simulink model "model_for_validation_bottom_section"  (R2022b)
settings: Solver=FixedStepAuto  StartTime=0.0  StopTime=5400  FixedStep=0.01  RelTol=1e-3
values from neighbouring files (symbols this model uses):
  A_bhp = area_cilinder    (= 0.006647610055)    [model_for_validation_bottom_section_script.m]
  A_bhp_air = A_thp_air    (= 0.0028902652413)    [model_for_validation_bottom_section_script.m]
  A_bi = area_cilinder    (= 0.006647610055)    [model_for_validation_bottom_section_script.m]
  A_bi_air = A_ti_air    (= 0.00578053048261)    [model_for_validation_bottom_section_script.m]
  A_bm = area_cilinder    (= 0.006647610055)    [model_for_validation_bottom_section_script.m]
  A_bm_air = A_tm_air    (= 0.0101159283446)    [model_for_validation_bottom_section_script.m]
  c_bc = c_tc    (= 460)    [model_for_validation_bottom_section_script.m]
  c_bhp = c_tm    (= 460)    [model_for_validation_bottom_section_script.m]
  c_bi = c_ti    (= 880)    [model_for_validation_bottom_section_script.m]
  c_bm = c_tm    (= 460)    [model_for_validation_bottom_section_script.m]
  D = 0    [model_for_validation_bottom_section_script.m]
  d_bhp = d_thp    (= 0.01)    [model_for_validation_bottom_section_script.m]
  d_bi = d_ti    (= 0.02)    [model_for_validation_bottom_section_script.m]
  d_bm = d_tm    (= 0.035)    [model_for_validation_bottom_section_script.m]
  h_c = 26.5    [model_for_validation_bottom_section_script.m]
  I = 0    [model_for_validation_bottom_section_script.m]
  k_bhp = k_tm    (= 22)    [model_for_validation_bottom_section_script.m]
  k_bi = k_ti    (= 0.3)    [model_for_validation_bottom_section_script.m]
  k_bm = k_tm    (= 22)    [model_for_validation_bottom_section_script.m]
  m_bc = m_tc    (= 0.0640332)    [model_for_validation_bottom_section_script.m]
  m_bhp = m_thp    (= 0.511865974235)    [model_for_validation_bottom_section_script.m]
  m_bi = m_ti    (= 0.29249484242)    [model_for_validation_bottom_section_script.m]
  m_bm = m_tm    (= 1.79153090982)    [model_for_validation_bottom_section_script.m]
  P = 100    [model_for_validation_bottom_section_script.m]
  P_rice = 1400    [model_for_validation_bottom_section_script.m]
  T_a = 18    [model_for_validation_bottom_section_script.m]
  T_init = T_a    (= 18)    [model_for_validation_bottom_section_script.m]
  T_setpoint = 285    [model_for_validation_bottom_section_script.m]
libraries: slpidlib x2, simulink x1
settings Model: PauseTimes=23  Creator=DLubbers  LastModifiedBy=DLubbers

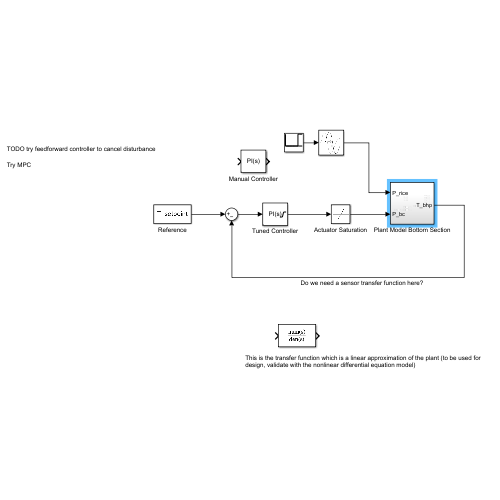
[thumbnail: Simulink's stored preview of the top-level diagram]
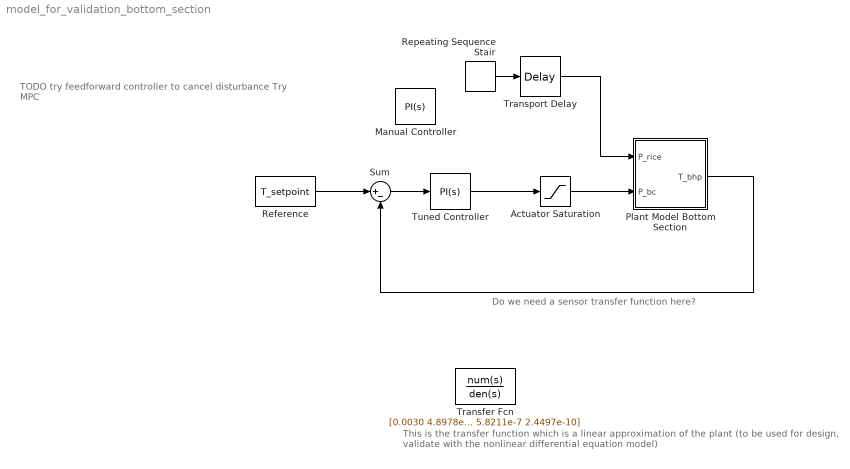
== system model_for_validation_bottom_section ==
  note: TODO try feedforward controller to cancel disturbance
      |
      | Try MPC
  note: This is the transfer function which is a linear approximation of the plant (to be used for design, validate with the nonlinear differential equation model)
  note: Do we need a sensor transfer function here?
  Actuator Saturation : Saturate  UpperLimit=690  LowerLimit=0
  Manual Controller : slpidlib/PID Controller  Controller=PI  Form=Parallel  TimeDomain=Continuous-time  UseExternalTs=off  SampleTime=-1  IntegratorMethod=Forward Euler  FilterMethod=Forward Euler  ControllerParametersSource=internal  P=P  I=I  UseKiTs=off  D=D  N=100  UseFilter=on  TunerSelectOption=Transfer Function Based (PID Tuner App)  InitialConditionSource=internal  InitialConditionForIntegrator=0  InitialConditionForFilter=0  DifferentiatorICPrevScaledInput=0  ExternalReset=none  TrackingMode=off  Kt=1  LimitOutput=off  SatLimitsSource=internal  UpperSaturationLimit=inf  LowerSaturationLimit=-inf  LinearizeAsGain=on  AntiWindupMode=none  Kb=1  LimitIntegrator=off  UpperIntegratorSaturationLimit=inf  LowerIntegratorSaturationLimit=-inf  POutMin=[]  POutMax=[]  IOutMin=[]  IOutMax=[]  DOutMin=[]  DOutMax=[]  NOutMin=[]  NOutMax=[]  SumOutMin=[]  SumOutMax=[]  SaturationOutMin=[]  SaturationOutMax=[]  PParamMin=[]  PParamMax=[]  IParamMin=[]  IParamMax=[]  DParamMin=[]  DParamMax=[]  NParamMin=[]  NParamMax=[]  KbParamMin=[]  KbParamMax=[]  KtParamMin=[]  KtParamMax=[]  KbOutMin=[]  KbOutMax=[]  KtOutMin=[]  KtOutMax=[]  IntegratorOutMin=[]  IntegratorOutMax=[]  FilterOutMin=[]  FilterOutMax=[]  SumI1OutMin=[]  SumI1OutMax=[]  SumI2OutMin=[]  SumI2OutMax=[]  SumI3OutMin=[]  SumI3OutMax=[]  SumI4OutMin=[]  SumI4OutMax=[]  SumDOutMin=[]  SumDOutMax=[]  DifferentiatorOutMin=[]  DifferentiatorOutMax=[]  FilterDiffOutCoefMin=[]  FilterDiffOutCoefMax=[]  ReciprocalOutMin=[]  ReciprocalOutMax=[]  SumDenOutMin=[]  SumDenOutMax=[]  SumNumOutMin=[]  SumNumOutMax=[]  DivideOutMin=[]  DivideOutMax=[]  UdiffTsProdOutMin=[]  UdiffTsProdOutMax=[]  NTsProdOutMin=[]  NTsProdOutMax=[]  UintegralTsProdOutMin=[]  UintegralTsProdOutMax=[]  UngainTsProdOutMin=[]  UngainTsProdOutMax=[]  ClampingZeroOutDataTypeStr=Inherit: Inherit via back propagation  ClampingZeroOutMin=[]  ClampingZeroOutMax=[]  FilterDenConstantOutDataTypeStr=Inherit: Inherit via back propagation  FilterDenConstantOutMin=[]  FilterDenConstantOutMax=[]  PCopyOutDataTypeStr=Inherit: Inherit via back propagation  PCopyOutMin=[]  PCopyOutMax=[]  NCopyOutDataTypeStr=Inherit: Inherit via back propagation  NCopyOutMin=[]  NCopyOutMax=[]  IntegratorContinuousStateAttributes=''  IntegratorStateMustResolveToSignalObject=off  IntegratorRTWStateStorageClass=Auto  FilterContinuousStateAttributes=''  FilterStateMustResolveToSignalObject=off  FilterRTWStateStorageClass=Auto  ParallelPVariant=InternalParameters  IdealPVariant=Disabled  IVariant=InternalParameters  DVariant=Disabled  IntegratorVariant=Continuous  SatVariant=Disabled  AWVariant=Passthrough  PCopyVariant=Disabled  TRVariant=Disabled  FdbkBlocksVariant=Forward  IdealPFdbkVariant=Disabled  SatFdbkVariant=Disabled  DerivativeFilterVariant=Disabled  NVariant=Disabled  NCopyVariant=Disabled_SignalSpec  FilterICVariant=Disabled  IntegratorICVariant=InternalICs  ExternalResetVariant=Disabled  TRSumVariant=Passthrough  SumFdbkVariant=Disabled  SumVariant=Sum_PI  TsampFilterVariant=InternalTs  TsampNgainVariant=Passthrough  TsampIntegralVariant=Passthrough  ExternalSaturationOutDataTypeStr=Inherit: Same as second input
  Plant Model Bottom Section : Subsystem
  Reference : Constant  Value=T_setpoint
  Repeating Sequence Stair : simulink/Sources/Repeating Sequence Stair  OutValues=[0 0 0 0 0 0 0 0 0 P_rice P_rice P_rice].'  tsamp=1  OutMin=[]  OutMax=[]  OutDataTypeStr=double  OutputDataTypeScalingMode=double  OutDataType=fixdt(0,8)  ConRadixGroup=Best Precision: Vector-wise  OutScaling=2^-12
  Sum : Sum  Inputs=|+-
  Transfer Fcn : TransferFcn  Numerator=[0.0030 4.8978e-5 2.5849e-7 4.3592e-10]  Denominator=[1 0.0288 2.3163e-4 5.8211e-7 2.4497e-10]
  Transport Delay : TransportDelay  DelayTime=3600
  Tuned Controller : slpidlib/PID Controller  Controller=PI  Form=Parallel  TimeDomain=Continuous-time  UseExternalTs=off  SampleTime=-1  IntegratorMethod=Forward Euler  FilterMethod=Forward Euler  ControllerParametersSource=internal  P=5.14299711444075  I=0.0389996474927596  UseKiTs=off  D=D  N=100  UseFilter=on  TunerSelectOption=Transfer Function Based (PID Tuner App)  InitialConditionSource=internal  InitialConditionForIntegrator=0  InitialConditionForFilter=0  DifferentiatorICPrevScaledInput=0  ExternalReset=none  TrackingMode=off  Kt=1  LimitOutput=on  SatLimitsSource=internal  UpperSaturationLimit=690  LowerSaturationLimit=0  LinearizeAsGain=on  AntiWindupMode=clamping  Kb=1  LimitIntegrator=off  UpperIntegratorSaturationLimit=inf  LowerIntegratorSaturationLimit=-inf  POutMin=[]  POutMax=[]  IOutMin=[]  IOutMax=[]  DOutMin=[]  DOutMax=[]  NOutMin=[]  NOutMax=[]  SumOutMin=[]  SumOutMax=[]  SaturationOutMin=[]  SaturationOutMax=[]  PParamMin=[]  PParamMax=[]  IParamMin=[]  IParamMax=[]  DParamMin=[]  DParamMax=[]  NParamMin=[]  NParamMax=[]  KbParamMin=[]  KbParamMax=[]  KtParamMin=[]  KtParamMax=[]  KbOutMin=[]  KbOutMax=[]  KtOutMin=[]  KtOutMax=[]  IntegratorOutMin=[]  IntegratorOutMax=[]  FilterOutMin=[]  FilterOutMax=[]  SumI1OutMin=[]  SumI1OutMax=[]  SumI2OutMin=[]  SumI2OutMax=[]  SumI3OutMin=[]  SumI3OutMax=[]  SumI4OutMin=[]  SumI4OutMax=[]  SumDOutMin=[]  SumDOutMax=[]  DifferentiatorOutMin=[]  DifferentiatorOutMax=[]  FilterDiffOutCoefMin=[]  FilterDiffOutCoefMax=[]  ReciprocalOutMin=[]  ReciprocalOutMax=[]  SumDenOutMin=[]  SumDenOutMax=[]  SumNumOutMin=[]  SumNumOutMax=[]  DivideOutMin=[]  DivideOutMax=[]  UdiffTsProdOutMin=[]  UdiffTsProdOutMax=[]  NTsProdOutMin=[]  NTsProdOutMax=[]  UintegralTsProdOutMin=[]  UintegralTsProdOutMax=[]  UngainTsProdOutMin=[]  UngainTsProdOutMax=[]  ClampingZeroOutDataTypeStr=Inherit: Inherit via back propagation  ClampingZeroOutMin=[]  ClampingZeroOutMax=[]  FilterDenConstantOutDataTypeStr=Inherit: Inherit via back propagation  FilterDenConstantOutMin=[]  FilterDenConstantOutMax=[]  PCopyOutDataTypeStr=Inherit: Inherit via back propagation  PCopyOutMin=[]  PCopyOutMax=[]  NCopyOutDataTypeStr=Inherit: Inherit via back propagation  NCopyOutMin=[]  NCopyOutMax=[]  IntegratorContinuousStateAttributes=''  IntegratorStateMustResolveToSignalObject=off  IntegratorRTWStateStorageClass=Auto  FilterContinuousStateAttributes=''  FilterStateMustResolveToSignalObject=off  FilterRTWStateStorageClass=Auto  ParallelPVariant=InternalParameters  IdealPVariant=Disabled  IVariant=InternalParameters  DVariant=Disabled  IntegratorVariant=Continuous  SatVariant=Enabled  AWVariant=ContClampingParallel  PCopyVariant=Disabled  TRVariant=Disabled  FdbkBlocksVariant=Forward  IdealPFdbkVariant=Disabled  SatFdbkVariant=Disabled  DerivativeFilterVariant=Disabled  NVariant=Disabled  NCopyVariant=Disabled_SignalSpec  FilterICVariant=Disabled  IntegratorICVariant=InternalICs  ExternalResetVariant=Disabled  TRSumVariant=Passthrough  SumFdbkVariant=Disabled  SumVariant=Sum_PI  TsampFilterVariant=InternalTs  TsampNgainVariant=Passthrough  TsampIntegralVariant=Passthrough  ExternalSaturationOutDataTypeStr=Inherit: Same as second input
  wires:
  Transport Delay/1 -> Plant Model Bottom Section/1(P_rice)
  Tuned Controller/1 -> Actuator Saturation/1
  Plant Model Bottom Section/1(T_bhp) -> Sum/2
  Sum/1 -> Tuned Controller/1
  Reference/1 -> Sum/1
  Actuator Saturation/1 -> Plant Model Bottom Section/2(P_bc)
  Repeating Sequence Stair/1 -> Transport Delay/1

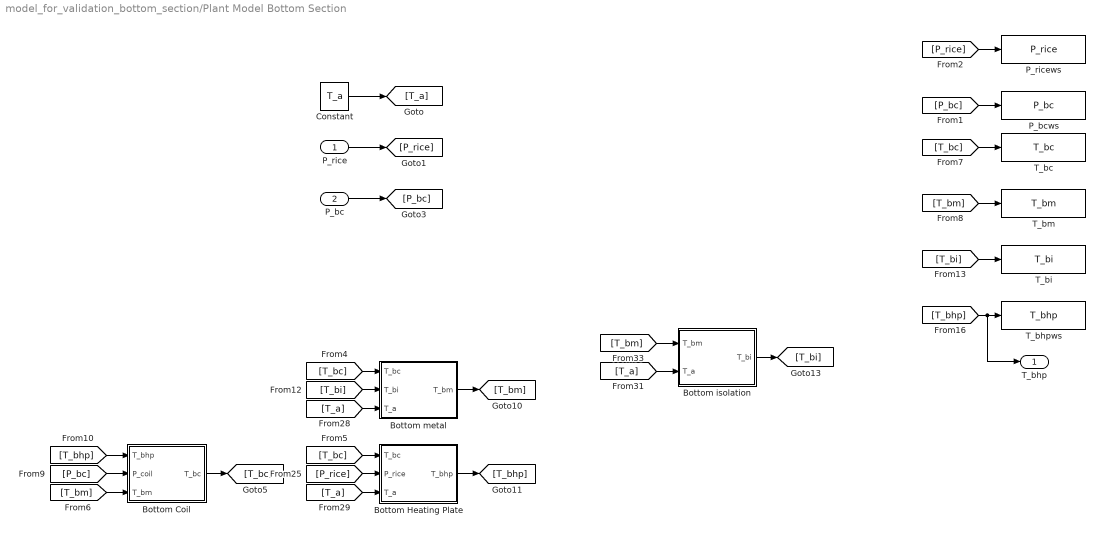
== system model_for_validation_bottom_section/Plant Model Bottom Section ==
  P_rice : Inport
  P_bc : Inport  Port=2
  Bottom Coil : Subsystem
  Bottom Heating Plate : Subsystem
  Bottom isolation : Subsystem
  Bottom metal : Subsystem
  Constant : Constant  Value=T_a
  P_bcws : ToWorkspace  VariableName=P_bc  SaveFormat=Timeseries  SampleTime=-1
  P_ricews : ToWorkspace  VariableName=P_rice  SaveFormat=Timeseries  SampleTime=-1
  T_bc : ToWorkspace  VariableName=T_bc  SaveFormat=Timeseries  SampleTime=-1
  T_bhpws : ToWorkspace  VariableName=T_bhp  SaveFormat=Timeseries  SampleTime=-1
  T_bi : ToWorkspace  VariableName=T_bi  SaveFormat=Timeseries  SampleTime=-1
  T_bm : ToWorkspace  VariableName=T_bm  SaveFormat=Timeseries  SampleTime=-1
  T_bhp : Outport
  wires:
  Constant/1 -> [T_a]
  [T_bhp] -> T_bhp/1, T_bhpws/1
  Bottom metal/1(T_bm) -> [T_bm]
  Bottom Coil/1(T_bc) -> [T_bc]
  [T_bc] -> Bottom metal/1(T_bc)
  [T_bi] -> T_bi/1
  [T_bm] -> Bottom isolation/1(T_bm)
  [T_a] -> Bottom Heating Plate/3(T_a)
  [T_a] -> Bottom metal/3(T_a)
  [T_bi] -> Bottom metal/2(T_bi)
  Bottom Heating Plate/1(T_bhp) -> [T_bhp]
  [T_bc] -> T_bc/1
  [T_a] -> Bottom isolation/2(T_a)
  [T_bhp] -> Bottom Coil/1(T_bhp)
  [T_bc] -> Bottom Heating Plate/1(T_bc)
  Bottom isolation/1(T_bi) -> [T_bi]
  [P_bc] -> Bottom Coil/2(P_coil)
  [P_rice] -> Bottom Heating Plate/2(P_rice)
  [T_bm] -> Bottom Coil/3(T_bm)
  [T_bm] -> T_bm/1
  P_bc/1 -> [P_bc]
  P_rice/1 -> [P_rice]
  [P_rice] -> P_ricews/1
  [P_bc] -> P_bcws/1

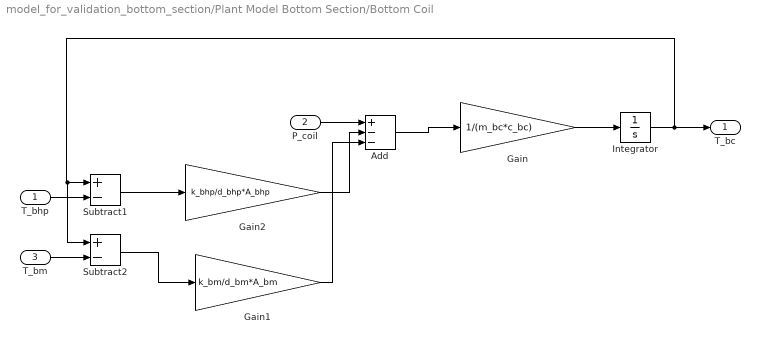
== system model_for_validation_bottom_section/Plant Model Bottom Section/Bottom Coil ==
  T_bhp : Inport
  P_coil : Inport  Port=2
  T_bm : Inport  Port=3
  Add : Sum  Inputs=+--
  Gain : Gain  Gain=1/(m_bc*c_bc)
  Gain1 : Gain  Gain=k_bm/d_bm*A_bm
  Gain2 : Gain  Gain=k_bhp/d_bhp*A_bhp
  Integrator : Integrator  InitialCondition=T_init
  Subtract1 : Sum  Inputs=+-
  Subtract2 : Sum  Inputs=+-
  T_bc : Outport
  wires:
  Gain/1 -> Integrator/1
  Add/1 -> Gain/1
  Subtract1/1 -> Gain2/1
  Gain2/1 -> Add/2
  T_bhp/1 -> Subtract1/2
  Integrator/1 -> T_bc/1, Subtract2/1, Subtract1/1
  P_coil/1 -> Add/1
  T_bm/1 -> Subtract2/2
  Subtract2/1 -> Gain1/1
  Gain1/1 -> Add/3

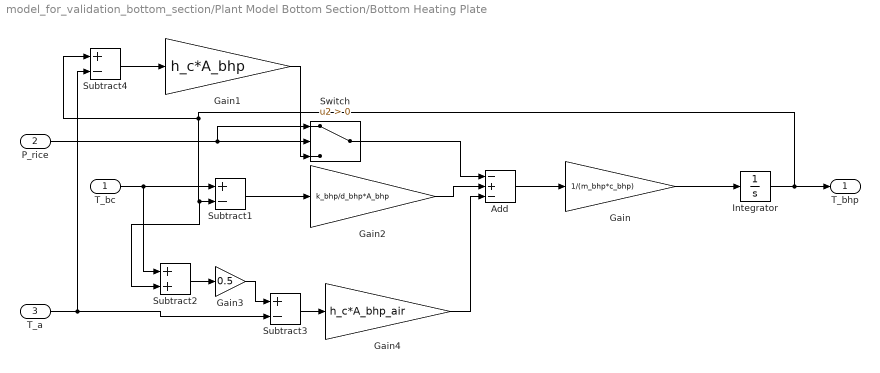
== system model_for_validation_bottom_section/Plant Model Bottom Section/Bottom Heating Plate ==
  T_bc : Inport
  P_rice : Inport  Port=2
  T_a : Inport  Port=3
  Add : Sum  Inputs=-+-
  Gain : Gain  Gain=1/(m_bhp*c_bhp)
  Gain1 : Gain  Gain=h_c*A_bhp
  Gain2 : Gain  Gain=k_bhp/d_bhp*A_bhp
  Gain3 : Gain  Gain=0.5
  Gain4 : Gain  Gain=h_c*A_bhp_air
  Integrator : Integrator  InitialCondition=T_init
  Subtract1 : Sum  Inputs=+-
  Subtract2 : Sum
  Subtract3 : Sum  Inputs=+-
  Subtract4 : Sum  Inputs=+-
  Switch : Switch  Criteria=u2 > Threshold  SaturateOnIntegerOverflow=off  InputSameDT=off
  T_bhp : Outport
  wires:
  P_rice/1 -> Switch/1, Switch/2
  Gain/1 -> Integrator/1
  Integrator/1 -> T_bhp/1, Subtract4/1, Subtract2/2, Subtract1/2
  Add/1 -> Gain/1
  Subtract1/1 -> Gain2/1
  T_bc/1 -> Subtract2/1, Subtract1/1
  Subtract3/1 -> Gain4/1
  T_a/1 -> Subtract4/2, Subtract3/2
  Subtract2/1 -> Gain3/1
  Gain3/1 -> Subtract3/1
  Gain2/1 -> Add/2
  Gain4/1 -> Add/3
  Switch/1 -> Add/1
  Gain1/1 -> Switch/3
  Subtract4/1 -> Gain1/1

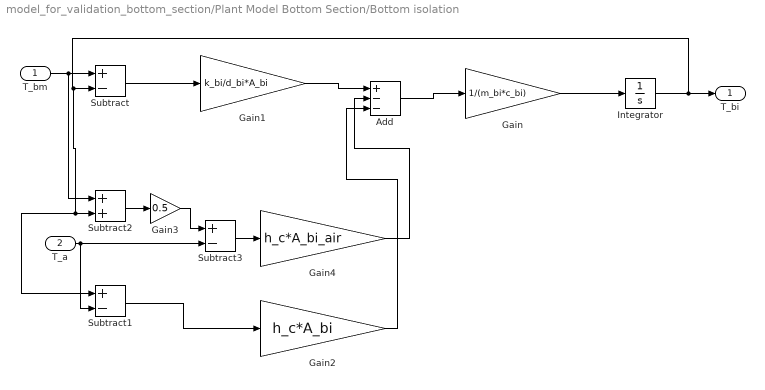
== system model_for_validation_bottom_section/Plant Model Bottom Section/Bottom isolation ==
  T_bm : Inport
  T_a : Inport  Port=2
  Add : Sum  Inputs=+--
  Gain : Gain  Gain=1/(m_bi*c_bi)
  Gain1 : Gain  Gain=k_bi/d_bi*A_bi
  Gain2 : Gain  Gain=h_c*A_bi
  Gain3 : Gain  Gain=0.5
  Gain4 : Gain  Gain=h_c*A_bi_air
  Integrator : Integrator  InitialCondition=T_init
  Subtract : Sum  Inputs=+-
  Subtract1 : Sum  Inputs=+-
  Subtract2 : Sum
  Subtract3 : Sum  Inputs=+-
  T_bi : Outport
  wires:
  Subtract/1 -> Gain1/1
  Gain/1 -> Integrator/1
  Add/1 -> Gain/1
  Integrator/1 -> Subtract2/2, Subtract1/1, Subtract/2, T_bi/1
  T_bm/1 -> Subtract2/1, Subtract/1
  Gain1/1 -> Add/1
  Subtract2/1 -> Gain3/1
  Gain3/1 -> Subtract3/1
  T_a/1 -> Subtract1/2, Subtract3/2
  Subtract3/1 -> Gain4/1
  Gain4/1 -> Add/2
  Gain2/1 -> Add/3
  Subtract1/1 -> Gain2/1

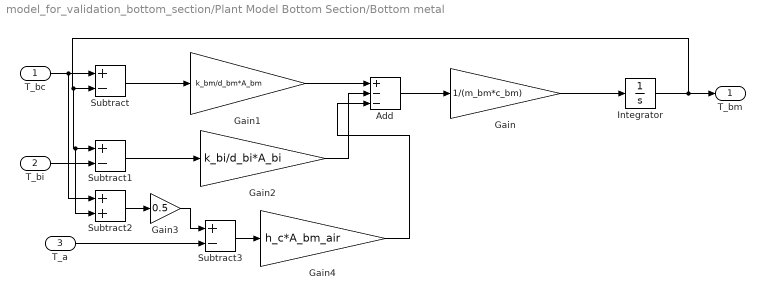
== system model_for_validation_bottom_section/Plant Model Bottom Section/Bottom metal ==
  T_bc : Inport
  T_bi : Inport  Port=2
  T_a : Inport  Port=3
  Add : Sum  Inputs=+--
  Gain : Gain  Gain=1/(m_bm*c_bm)
  Gain1 : Gain  Gain=k_bm/d_bm*A_bm
  Gain2 : Gain  Gain=k_bi/d_bi*A_bi
  Gain3 : Gain  Gain=0.5
  Gain4 : Gain  Gain=h_c*A_bm_air
  Integrator : Integrator  InitialCondition=T_init
  Subtract : Sum  Inputs=+-
  Subtract1 : Sum  Inputs=+-
  Subtract2 : Sum
  Subtract3 : Sum  Inputs=+-
  T_bm : Outport
  wires:
  Subtract/1 -> Gain1/1
  Gain/1 -> Integrator/1
  Add/1 -> Gain/1
  Subtract1/1 -> Gain2/1
  T_bi/1 -> Subtract1/2
  Integrator/1 -> Subtract2/2, Subtract1/1, Subtract/2, T_bm/1
  T_bc/1 -> Subtract2/1, Subtract/1
  Gain1/1 -> Add/1
  Gain2/1 -> Add/2
  Subtract2/1 -> Gain3/1
  Gain3/1 -> Subtract3/1
  T_a/1 -> Subtract3/2
  Subtract3/1 -> Gain4/1
  Gain4/1 -> Add/3
